simulink subsystem "SimscapePlantModels"  (R2023b)
settings: Solver=VariableStepAuto  StartTime=0.0  StopTime=10.0  RelTol=1e-3
undefined symbols (not defined in the file or in its folder): AxlFL, AxlFR, AxlRL, AxlRR, PlntTrnsfrCaseAxlSpdLock, PlntTrnsfrCaseTrqSplitRatio
libraries: fl_lib x13, nesl_utility_internal x9, sdl_lib x3, simulink x2, nesl_utility x2
(part 2 of 2)

== system SimscapePlantModels/Drivetrain/Drivetrain Layout/AxlTrqRL ==
  Ideal Torque Sensor : fl_lib/Mechanical/Mechanical Sensors/Ideal Torque Sensor
  PS-Simulink Converter : nesl_utility_internal/PS-Simulink Converter  PhysicalDomain=network_engine_domain  SubClassName=ps_output  LeftPortType=input  RightPortType=output  PseudoPeriodic=off  Frequencies=[]  VectorFormat=inherit  Unit=inherit  AffineConversion=off
  R : PMIOPort  Side=Left
  C : PMIOPort  Port=2  Side=Right
  Trq : Outport
  wires:
  PS-Simulink Converter/1 -> Trq/1
  connections:
  Ideal Torque Sensor/LConn1 -- R/RConn1
  Ideal Torque Sensor/RConn1 -- C/RConn1
  PS-Simulink Converter/LConn1 -- Ideal Torque Sensor/RConn2

== system SimscapePlantModels/Drivetrain/Drivetrain Layout/Axle Interconnect ==
  SplitRatio : Inport
  Lockup : Inport  Port=2
  NoInterconnectSSC : Subsystem  VariantControl=NoInterconnectSSC  ReferencedSubsystem=NoInterconnectSSC
  TransferCaseSSC : Subsystem  VariantControl=TransferCaseSSC  ReferencedSubsystem=TransferCaseSSC
  FrntDiffrntlTrq : PMIOPort  Side=Left
  DriveshftTrq : PMIOPort  Port=2  Side=Left
  RearDiffrntlTrq : PMIOPort  Port=3  Side=Left

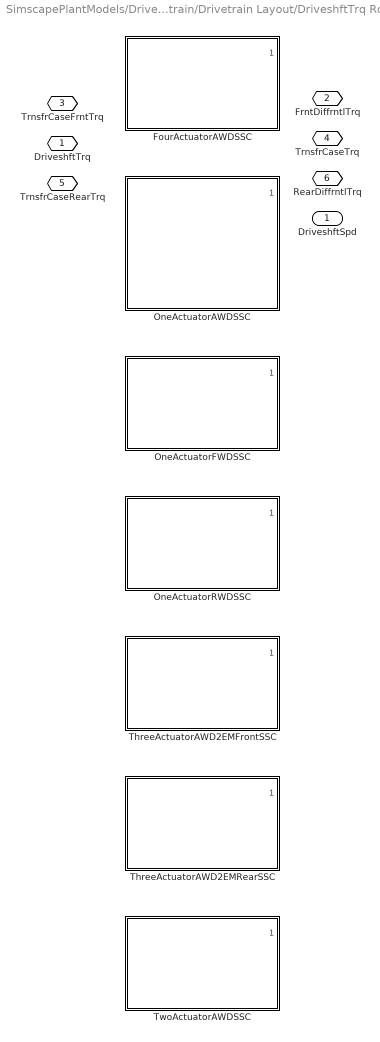
== system SimscapePlantModels/Drivetrain/Drivetrain Layout/DriveshftTrq Routing ==
  FourActuatorAWDSSC : Subsystem  VariantControl=FourActuatorAWDSSC  ReferencedSubsystem=FourActuatorAWDSSC
  OneActuatorAWDSSC : Subsystem  VariantControl=OneActuatorAWDSSC  ReferencedSubsystem=OneActuatorAWDSSC
  OneActuatorFWDSSC : Subsystem  VariantControl=OneActuatorFWDSSC  ReferencedSubsystem=OneActuatorFWDSSC
  OneActuatorRWDSSC : Subsystem  VariantControl=OneActuatorRWDSSC  ReferencedSubsystem=OneActuatorRWDSSC
  ThreeActuatorAWD2EMFrontSSC : Subsystem  VariantControl=ThreeActuatorAWD2EMFrontSSC  ReferencedSubsystem=ThreeActuatorAWD2EMFrontSSC
  ThreeActuatorAWD2EMRearSSC : Subsystem  VariantControl=ThreeActuatorAWD2EMRearSSC  ReferencedSubsystem=ThreeActuatorAWD2EMRearSSC
  TwoActuatorAWDSSC : Subsystem  VariantControl=TwoActuatorAWDSSC  ReferencedSubsystem=TwoActuatorAWDSSC
  DriveshftTrq : PMIOPort  Side=Left
  FrntDiffrntlTrq : PMIOPort  Port=2  Side=Right
  TrnsfrCaseFrntTrq : PMIOPort  Port=3  Side=Right
  TrnsfrCaseTrq : PMIOPort  Port=4  Side=Right
  TrnsfrCaseRearTrq : PMIOPort  Port=5  Side=Right
  RearDiffrntlTrq : PMIOPort  Port=6  Side=Right
  DriveshftSpd : Outport  VectorParamsAs1DForOutWhenUnconnected=off

== system SimscapePlantModels/Drivetrain/Drivetrain Layout/Front Axle ==
  Prs1 : Inport
  Prs2 : Inport  Port=2
  DualEMDriveFrontSSC : Subsystem  VariantControl=DualEMDriveFrontSSC  ReferencedSubsystem=DualEMDriveFrontSSC
  LimitedSlipDifferentialSSC : Subsystem  VariantControl=LimitedSlipDifferentialSSC  ReferencedSubsystem=LimitedSlipDifferentialSSC
  NoDifferentialFrontSSC : Subsystem  VariantControl=NoDifferentialFrontSSC  ReferencedSubsystem=NoDifferentialFrontSSC
  OpenDifferentialSSC : Subsystem  VariantControl=OpenDifferentialSSC  ReferencedSubsystem=OpenDifferentialSSC
  DriveshftTrq : PMIOPort  Side=Left
  AxlTrqFL : PMIOPort  Port=2  Side=Right
  AxlTrqFR : PMIOPort  Port=3  Side=Right
  Info : Outport
  DriveshftSpd : Outport  Port=2
  Axl1Spd : Outport  Port=3
  Axl2Spd : Outport  Port=4

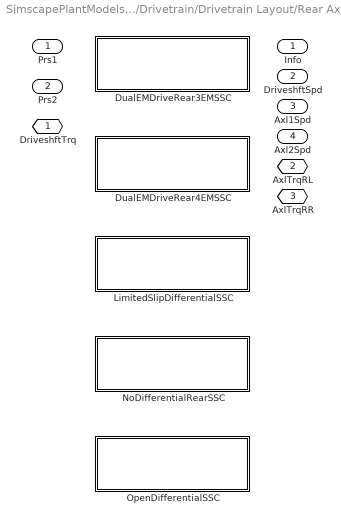
== system SimscapePlantModels/Drivetrain/Drivetrain Layout/Rear Axle ==
  Prs1 : Inport
  Prs2 : Inport  Port=2
  DualEMDriveRear3EMSSC : Subsystem  VariantControl=DualEMDriveRear3EMSSC  ReferencedSubsystem=DualEMDriveRear3EMSSC
  DualEMDriveRear4EMSSC : Subsystem  VariantControl=DualEMDriveRear4EMSSC  ReferencedSubsystem=DualEMDriveRear4EMSSC
  LimitedSlipDifferentialSSC : Subsystem  VariantControl=LimitedSlipDifferentialSSC  ReferencedSubsystem=LimitedSlipDifferentialSSC
  NoDifferentialRearSSC : Subsystem  VariantControl=NoDifferentialRearSSC  ReferencedSubsystem=NoDifferentialRearSSC
  OpenDifferentialSSC : Subsystem  VariantControl=OpenDifferentialSSC  ReferencedSubsystem=OpenDifferentialSSC
  DriveshftTrq : PMIOPort  Side=Left
  AxlTrqRL : PMIOPort  Port=2  Side=Right
  AxlTrqRR : PMIOPort  Port=3  Side=Right
  Info : Outport
  DriveshftSpd : Outport  Port=2
  Axl1Spd : Outport  Port=3
  Axl2Spd : Outport  Port=4
